simulink model "diagram"  (R2022a)
settings: Solver=VariableStepAuto  StartTime=0.0  StopTime=10.0  RelTol=1e-3
settings Model: Creator=tomsl  LastModifiedBy=tomsl

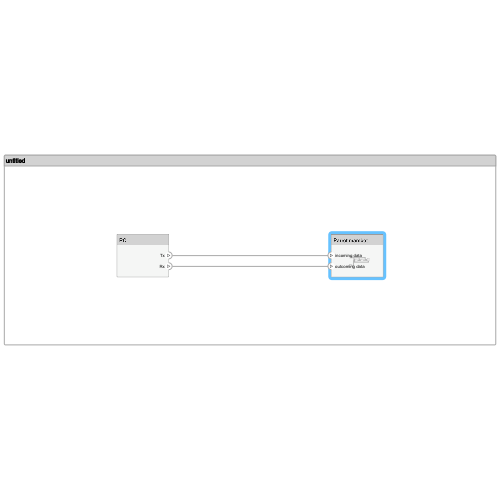
[thumbnail: Simulink's stored preview of the top-level diagram]
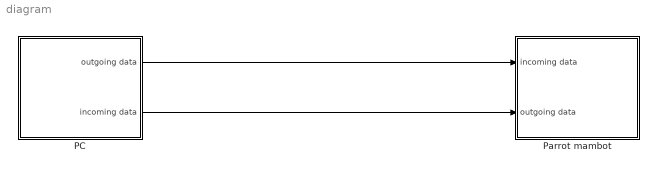
== system diagram ==
  PC : Subsystem
      settings: PortSchema="{\"entries\":[{\"content\":{\"headerSize\":26,\"margin\":15,\"minimumSpacing\":25,\"sides\":[{\"content\":{\"connectorIds\":[]},\"type\":\"ConnectorPlacement.EquallySpacedRectSide\",\"uuid\":\"57f66509-e8d0-4a15-b15f-6e72d08a95fa\"},{\"content\":{\"connectorIds\":[\"Out1\",\"Out2\"],\"side\":\"RIGHT\"},\"type\":\"ConnectorPlacement.EquallySpacedRectSide\",\"uuid\":\"4d6ddc62-5d39-4aa3-bc43-22ec2045b1a1\"},{\"content\":{\"connectorIds\":[],\"side\":\"TOP\"},\"type\":\"ConnectorPlacement.EquallySpacedRectSide\",\"uuid\":\"3f7e3717-be44-4e9b-bb5f-b3098bc3e8c0\"}]},\"type\":\"ConnectorPlacement.EquallySpacedConnector\",\"uuid\":\"3e666d01-11f0-4990-a987-17249c891680\"}],\"packageUris\":[\"http://schema.mathworks.com/mf0/Connector/R2020b\"],\"version\":\"1.0\"}"
  Parrot mambot : Subsystem
      settings: PortSchema="{\"entries\":[{\"content\":{\"headerSize\":26,\"margin\":15,\"minimumSpacing\":25,\"sides\":[{\"content\":{\"connectorIds\":[\"In1\",\"In2\"]},\"type\":\"ConnectorPlacement.EquallySpacedRectSide\",\"uuid\":\"57f66509-e8d0-4a15-b15f-6e72d08a95fa\"},{\"content\":{\"connectorIds\":[],\"side\":\"RIGHT\"},\"type\":\"ConnectorPlacement.EquallySpacedRectSide\",\"uuid\":\"4d6ddc62-5d39-4aa3-bc43-22ec2045b1a1\"},{\"content\":{\"connectorIds\":[],\"side\":\"TOP\"},\"type\":\"ConnectorPlacement.EquallySpacedRectSide\",\"uuid\":\"3f7e3717-be44-4e9b-bb5f-b3098bc3e8c0\"}]},\"type\":\"ConnectorPlacement.EquallySpacedConnector\",\"uuid\":\"3e666d01-11f0-4990-a987-17249c891680\"}],\"packageUris\":[\"http://schema.mathworks.com/mf0/Connector/R2020b\"],\"version\":\"1.0\"}"
  wires:
  PC/1(outgoing data) -> Parrot mambot/1(incoming data)
  PC/2(incoming data) -> Parrot mambot/2(outgoing data)

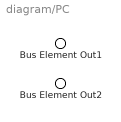
== system diagram/PC ==
  Bus Element Out1 : Outport  PortName=outgoing data
  Bus Element Out2 : Outport  Port=2  PortName=incoming data

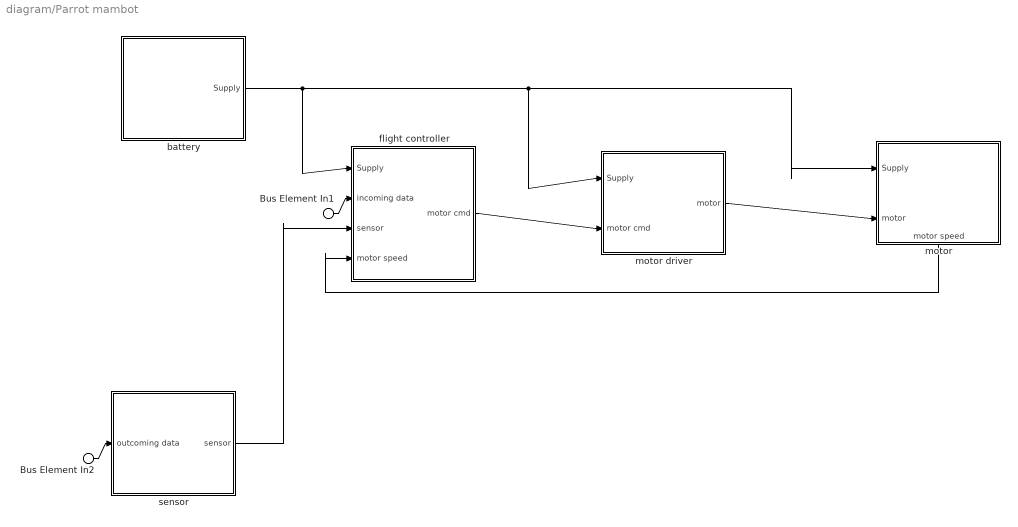
== system diagram/Parrot mambot ==
  Bus Element In1 : Inport  PortName=incoming data
  Bus Element In2 : Inport  Port=2  PortName=outgoing data
  battery : Subsystem
      settings: PortSchema="{\"entries\":[{\"content\":{\"headerSize\":26,\"margin\":15,\"minimumSpacing\":25,\"sides\":[{\"content\":{\"connectorIds\":[]},\"type\":\"ConnectorPlacement.EquallySpacedRectSide\",\"uuid\":\"57f66509-e8d0-4a15-b15f-6e72d08a95fa\"},{\"content\":{\"connectorIds\":[\"Out1\"],\"side\":\"RIGHT\"},\"type\":\"ConnectorPlacement.EquallySpacedRectSide\",\"uuid\":\"4d6ddc62-5d39-4aa3-bc43-22ec2045b1a1\"},{\"content\":{\"connectorIds\":[],\"side\":\"TOP\"},\"type\":\"ConnectorPlacement.EquallySpacedRectSide\",\"uuid\":\"3f7e3717-be44-4e9b-bb5f-b3098bc3e8c0\"}]},\"type\":\"ConnectorPlacement.EquallySpacedConnector\",\"uuid\":\"3e666d01-11f0-4990-a987-17249c891680\"}],\"packageUris\":[\"http://schema.mathworks.com/mf0/Connector/R2020b\"],\"version\":\"1.0\"}"
  flight controller : Subsystem
      settings: PortSchema="{\"entries\":[{\"content\":{\"headerSize\":26,\"margin\":15,\"minimumSpacing\":25,\"sides\":[{\"content\":{\"connectorIds\":[\"In1\",\"In2\",\"In3\",\"In4\"]},\"type\":\"ConnectorPlacement.EquallySpacedRectSide\",\"uuid\":\"57f66509-e8d0-4a15-b15f-6e72d08a95fa\"},{\"content\":{\"connectorIds\":[\"Out1\"],\"side\":\"RIGHT\"},\"type\":\"ConnectorPlacement.EquallySpacedRectSide\",\"uuid\":\"4d6ddc62-5d39-4aa3-bc43-22ec2045b1a1\"},{\"content\":{\"connectorIds\":[],\"side\":\"TOP\"},\"type\":\"ConnectorPlacement.EquallySpacedRectSide\",\"uuid\":\"3f7e3717-be44-4e9b-bb5f-b3098bc3e8c0\"}]},\"type\":\"ConnectorPlacement.EquallySpacedConnector\",\"uuid\":\"3e666d01-11f0-4990-a987-17249c891680\"}],\"packageUris\":[\"http://schema.mathworks.com/mf0/Connector/R2020b\"],\"version\":\"1.0\"}"
  motor : Subsystem
      settings: PortSchema="{\"entries\":[{\"content\":{\"headerSize\":26,\"margin\":15,\"minimumSpacing\":25,\"sides\":[{\"content\":{\"connectorIds\":[\"In1\",\"In2\"]},\"type\":\"ConnectorPlacement.EquallySpacedRectSide\",\"uuid\":\"57f66509-e8d0-4a15-b15f-6e72d08a95fa\"},{\"content\":{\"connectorIds\":[],\"side\":\"RIGHT\"},\"type\":\"ConnectorPlacement.EquallySpacedRectSide\",\"uuid\":\"4d6ddc62-5d39-4aa3-bc43-22ec2045b1a1\"},{\"content\":{\"connectorIds\":[],\"side\":\"TOP\"},\"type\":\"ConnectorPlacement.EquallySpacedRectSide\",\"uuid\":\"3f7e3717-be44-4e9b-bb5f-b3098bc3e8c0\"},{\"content\":{\"connectorIds\":[\"Out1\"],\"side\":\"BOTTOM\"},\"type\":\"ConnectorPlacement.EquallySpacedRectSide\",\"uuid\":\"6960d807-46f0-4522-a601-ab1e5094de18\"}]},\"type\":\"ConnectorPlacement.EquallySpacedConnector\",\"uuid\":\"3e666d01-11f0-4990-a987-17249c891680\"}],\"packageUris\":[\"http://schema.mathworks.com/mf0/Connector/R2020b\"],\"version\":\"1.0\"}"
  motor driver : Subsystem
      settings: PortSchema="{\"entries\":[{\"content\":{\"headerSize\":26,\"margin\":15,\"minimumSpacing\":25,\"sides\":[{\"content\":{\"connectorIds\":[\"In1\",\"In2\"]},\"type\":\"ConnectorPlacement.EquallySpacedRectSide\",\"uuid\":\"57f66509-e8d0-4a15-b15f-6e72d08a95fa\"},{\"content\":{\"connectorIds\":[\"Out1\"],\"side\":\"RIGHT\"},\"type\":\"ConnectorPlacement.EquallySpacedRectSide\",\"uuid\":\"4d6ddc62-5d39-4aa3-bc43-22ec2045b1a1\"},{\"content\":{\"connectorIds\":[],\"side\":\"TOP\"},\"type\":\"ConnectorPlacement.EquallySpacedRectSide\",\"uuid\":\"3f7e3717-be44-4e9b-bb5f-b3098bc3e8c0\"}]},\"type\":\"ConnectorPlacement.EquallySpacedConnector\",\"uuid\":\"3e666d01-11f0-4990-a987-17249c891680\"}],\"packageUris\":[\"http://schema.mathworks.com/mf0/Connector/R2020b\"],\"version\":\"1.0\"}"
  sensor : Subsystem
      settings: PortSchema="{\"entries\":[{\"content\":{\"headerSize\":26,\"margin\":15,\"minimumSpacing\":25,\"sides\":[{\"content\":{\"connectorIds\":[\"In1\"]},\"type\":\"ConnectorPlacement.EquallySpacedRectSide\",\"uuid\":\"57f66509-e8d0-4a15-b15f-6e72d08a95fa\"},{\"content\":{\"connectorIds\":[\"Out1\"],\"side\":\"RIGHT\"},\"type\":\"ConnectorPlacement.EquallySpacedRectSide\",\"uuid\":\"4d6ddc62-5d39-4aa3-bc43-22ec2045b1a1\"},{\"content\":{\"connectorIds\":[],\"side\":\"TOP\"},\"type\":\"ConnectorPlacement.EquallySpacedRectSide\",\"uuid\":\"3f7e3717-be44-4e9b-bb5f-b3098bc3e8c0\"}]},\"type\":\"ConnectorPlacement.EquallySpacedConnector\",\"uuid\":\"3e666d01-11f0-4990-a987-17249c891680\"}],\"packageUris\":[\"http://schema.mathworks.com/mf0/Connector/R2020b\"],\"version\":\"1.0\"}"
  wires:
  Bus Element In1/1 -> flight controller/2(incoming data)
  Bus Element In2/1 -> sensor/1(outcoming data)
  motor driver/1(motor) -> motor/2(motor)
  sensor/1(sensor) -> flight controller/3(sensor)
  flight controller/1(motor cmd) -> motor driver/2(motor cmd)
  motor/1(motor speed) -> flight controller/4(motor speed)
  battery/1(Supply) -> motor/1(Supply), motor driver/1(Supply), flight controller/1(Supply)

== system diagram/Parrot mambot/battery ==
  Bus Element Out1 : Outport  PortName=Supply

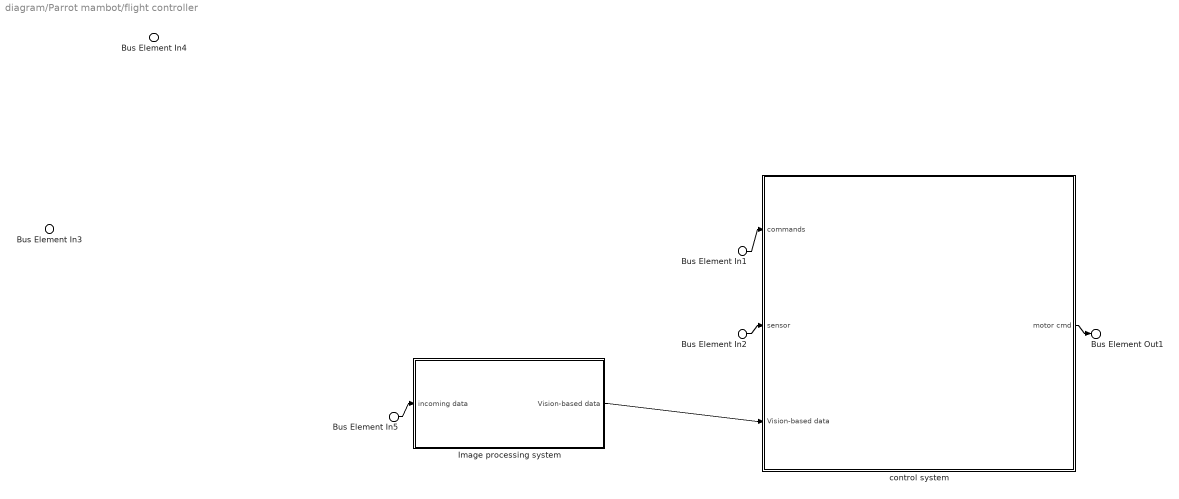
== system diagram/Parrot mambot/flight controller ==
  Bus Element In4 : Inport  PortName=Supply
  Bus Element In1 : Inport  Port=2  PortName=incoming data
  Bus Element In5 : Inport  Port=2  PortName=incoming data
  Bus Element In2 : Inport  Port=3  PortName=sensor
  Bus Element In3 : Inport  Port=4  PortName=motor speed
  Image processing system : Subsystem
      settings: PortSchema="{\"entries\":[{\"content\":{\"headerSize\":26,\"margin\":15,\"minimumSpacing\":25,\"sides\":[{\"content\":{\"connectorIds\":[\"In1\"]},\"type\":\"ConnectorPlacement.EquallySpacedRectSide\",\"uuid\":\"57f66509-e8d0-4a15-b15f-6e72d08a95fa\"},{\"content\":{\"connectorIds\":[\"Out1\"],\"side\":\"RIGHT\"},\"type\":\"ConnectorPlacement.EquallySpacedRectSide\",\"uuid\":\"4d6ddc62-5d39-4aa3-bc43-22ec2045b1a1\"},{\"content\":{\"connectorIds\":[],\"side\":\"TOP\"},\"type\":\"ConnectorPlacement.EquallySpacedRectSide\",\"uuid\":\"3f7e3717-be44-4e9b-bb5f-b3098bc3e8c0\"}]},\"type\":\"ConnectorPlacement.EquallySpacedConnector\",\"uuid\":\"3e666d01-11f0-4990-a987-17249c891680\"}],\"packageUris\":[\"http://schema.mathworks.com/mf0/Connector/R2020b\"],\"version\":\"1.0\"}"
  control system : Subsystem
      settings: PortSchema="{\"entries\":[{\"content\":{\"headerSize\":26,\"margin\":15,\"minimumSpacing\":25,\"sides\":[{\"content\":{\"connectorIds\":[\"In1\",\"In2\",\"In3\"]},\"type\":\"ConnectorPlacement.EquallySpacedRectSide\",\"uuid\":\"57f66509-e8d0-4a15-b15f-6e72d08a95fa\"},{\"content\":{\"connectorIds\":[\"Out1\"],\"side\":\"RIGHT\"},\"type\":\"ConnectorPlacement.EquallySpacedRectSide\",\"uuid\":\"4d6ddc62-5d39-4aa3-bc43-22ec2045b1a1\"},{\"content\":{\"connectorIds\":[],\"side\":\"TOP\"},\"type\":\"ConnectorPlacement.EquallySpacedRectSide\",\"uuid\":\"3f7e3717-be44-4e9b-bb5f-b3098bc3e8c0\"}]},\"type\":\"ConnectorPlacement.EquallySpacedConnector\",\"uuid\":\"3e666d01-11f0-4990-a987-17249c891680\"}],\"packageUris\":[\"http://schema.mathworks.com/mf0/Connector/R2020b\"],\"version\":\"1.0\"}"
  Bus Element Out1 : Outport  PortName=motor cmd
  wires:
  Image processing system/1(Vision-based data) -> control system/3(Vision-based data)
  Bus Element In2/1 -> control system/2(sensor)
  Bus Element In1/1 -> control system/1(commands)
  Bus Element In5/1 -> Image processing system/1(incoming data)
  control system/1(motor cmd) -> Bus Element Out1/1

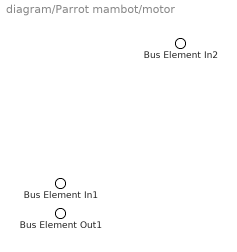
== system diagram/Parrot mambot/motor ==
  Bus Element In2 : Inport  PortName=Supply
  Bus Element In1 : Inport  Port=2  PortName=motor
  Bus Element Out1 : Outport  PortName=motor speed

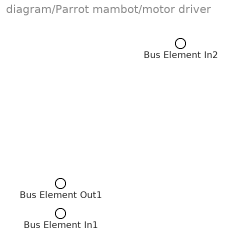
== system diagram/Parrot mambot/motor driver ==
  Bus Element In2 : Inport  PortName=Supply
  Bus Element In1 : Inport  Port=2  PortName=motor cmd
  Bus Element Out1 : Outport  PortName=motor

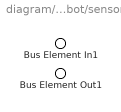
== system diagram/Parrot mambot/sensor ==
  Bus Element In1 : Inport  PortName=outcoming data
  Bus Element Out1 : Outport  PortName=sensor

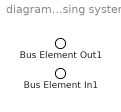
== system diagram/Parrot mambot/flight controller/Image processing system ==
  Bus Element In1 : Inport  PortName=incoming data
  Bus Element Out1 : Outport  PortName=Vision-based data

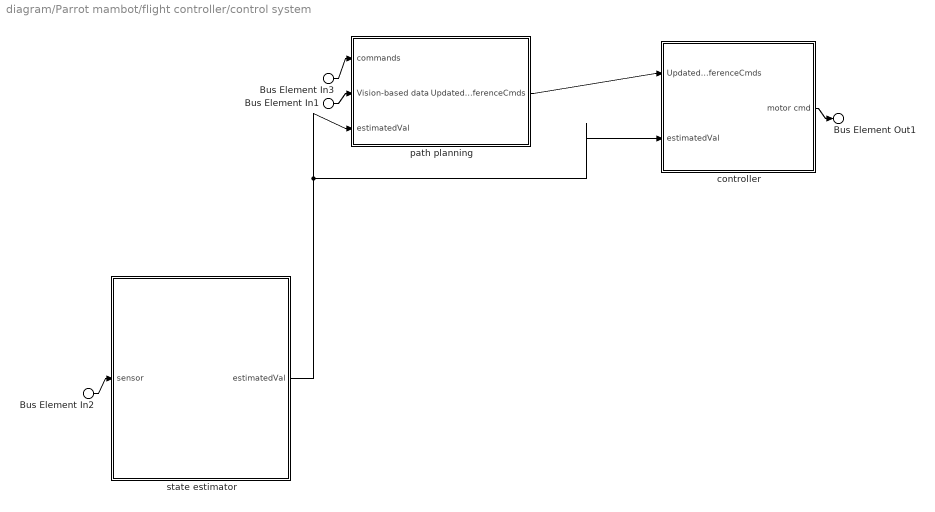
== system diagram/Parrot mambot/flight controller/control system ==
  Bus Element In3 : Inport  PortName=commands
  Bus Element In2 : Inport  Port=2  PortName=sensor
  Bus Element In1 : Inport  Port=3  PortName=Vision-based data
  controller : Subsystem
      settings: PortSchema="{\"entries\":[{\"content\":{\"headerSize\":26,\"margin\":15,\"minimumSpacing\":25,\"sides\":[{\"content\":{\"connectorIds\":[\"In1\",\"In2\"]},\"type\":\"ConnectorPlacement.EquallySpacedRectSide\",\"uuid\":\"57f66509-e8d0-4a15-b15f-6e72d08a95fa\"},{\"content\":{\"connectorIds\":[\"Out1\"],\"side\":\"RIGHT\"},\"type\":\"ConnectorPlacement.EquallySpacedRectSide\",\"uuid\":\"4d6ddc62-5d39-4aa3-bc43-22ec2045b1a1\"},{\"content\":{\"connectorIds\":[],\"side\":\"TOP\"},\"type\":\"ConnectorPlacement.EquallySpacedRectSide\",\"uuid\":\"3f7e3717-be44-4e9b-bb5f-b3098bc3e8c0\"}]},\"type\":\"ConnectorPlacement.EquallySpacedConnector\",\"uuid\":\"3e666d01-11f0-4990-a987-17249c891680\"}],\"packageUris\":[\"http://schema.mathworks.com/mf0/Connector/R2020b\"],\"version\":\"1.0\"}"
  path planning : Subsystem
      settings: PortSchema="{\"entries\":[{\"content\":{\"headerSize\":26,\"margin\":15,\"minimumSpacing\":25,\"sides\":[{\"content\":{\"connectorIds\":[\"In1\",\"In2\",\"In3\"]},\"type\":\"ConnectorPlacement.EquallySpacedRectSide\",\"uuid\":\"57f66509-e8d0-4a15-b15f-6e72d08a95fa\"},{\"content\":{\"connectorIds\":[\"Out1\"],\"side\":\"RIGHT\"},\"type\":\"ConnectorPlacement.EquallySpacedRectSide\",\"uuid\":\"4d6ddc62-5d39-4aa3-bc43-22ec2045b1a1\"},{\"content\":{\"connectorIds\":[],\"side\":\"TOP\"},\"type\":\"ConnectorPlacement.EquallySpacedRectSide\",\"uuid\":\"3f7e3717-be44-4e9b-bb5f-b3098bc3e8c0\"}]},\"type\":\"ConnectorPlacement.EquallySpacedConnector\",\"uuid\":\"3e666d01-11f0-4990-a987-17249c891680\"}],\"packageUris\":[\"http://schema.mathworks.com/mf0/Connector/R2020b\"],\"version\":\"1.0\"}"
  state estimator : Subsystem
      settings: PortSchema="{\"entries\":[{\"content\":{\"headerSize\":26,\"margin\":15,\"minimumSpacing\":25,\"sides\":[{\"content\":{\"connectorIds\":[\"In1\"]},\"type\":\"ConnectorPlacement.EquallySpacedRectSide\",\"uuid\":\"57f66509-e8d0-4a15-b15f-6e72d08a95fa\"},{\"content\":{\"connectorIds\":[\"Out1\"],\"side\":\"RIGHT\"},\"type\":\"ConnectorPlacement.EquallySpacedRectSide\",\"uuid\":\"4d6ddc62-5d39-4aa3-bc43-22ec2045b1a1\"},{\"content\":{\"connectorIds\":[],\"side\":\"TOP\"},\"type\":\"ConnectorPlacement.EquallySpacedRectSide\",\"uuid\":\"3f7e3717-be44-4e9b-bb5f-b3098bc3e8c0\"}]},\"type\":\"ConnectorPlacement.EquallySpacedConnector\",\"uuid\":\"3e666d01-11f0-4990-a987-17249c891680\"}],\"packageUris\":[\"http://schema.mathworks.com/mf0/Connector/R2020b\"],\"version\":\"1.0\"}"
  Bus Element Out1 : Outport  PortName=motor cmd
  wires:
  Bus Element In1/1 -> path planning/2(Vision-based data)
  Bus Element In2/1 -> state estimator/1(sensor)
  state estimator/1(estimatedVal) -> controller/2(estimatedVal), path planning/3(estimatedVal)
  Bus Element In3/1 -> path planning/1(commands)
  path planning/1(UpdatedReferenceCmds) -> controller/1(UpdatedReferenceCmds)
  controller/1(motor cmd) -> Bus Element Out1/1

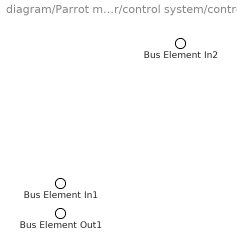
== system diagram/Parrot mambot/flight controller/control system/controller ==
  Bus Element In2 : Inport  PortName=UpdatedReferenceCmds
  Bus Element In1 : Inport  Port=2  PortName=estimatedVal
  Bus Element Out1 : Outport  PortName=motor cmd

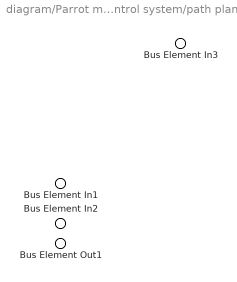
== system diagram/Parrot mambot/flight controller/control system/path planning ==
  Bus Element In3 : Inport  PortName=commands
  Bus Element In1 : Inport  Port=2  PortName=Vision-based data
  Bus Element In2 : Inport  Port=3  PortName=estimatedVal
  Bus Element Out1 : Outport  PortName=UpdatedReferenceCmds

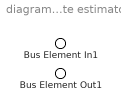
== system diagram/Parrot mambot/flight controller/control system/state estimator ==
  Bus Element In1 : Inport  PortName=sensor
  Bus Element Out1 : Outport  PortName=estimatedVal
